simulink model "Simulation_Fahrmodell_v4_straight_line_v1"  (R2023b)
settings: Solver=ode14x  StartTime=0.0  StopTime=500  FixedStep=0.005  RelTol=1e-3
undefined symbols (not defined in the file): bat, cp, cp_Zelle_JpkgK, gb, Ice_derfacLoadDecrease_MAP, Ice_derfacLoadIncrease_MAP, Ice_n_axis, Ice_relLoadMax_CUR_n, Ice_relLoadMax_CUR_val, Ice_rl_axis_norm, P4, P4_DM, pt, seconds, SKO_STREET_CHAL, SKO_WHEEL_TYP_CHAL, slip_pacejka, T_init_degC, Track, TT_sliced, use_turbo_model, v_Fzg_init_kmph, veh
libraries: nesl_utility x15, fl_lib x9, simulink x4
(part 4 of 7)

== system Simulation_Fahrmodell_v4_straight_line_v1/Vehicle Dynamics Model /Drivetrain/GETRIEBE auswahl VK, EV/Transmission Selector1/ICE Multi-Speed/Simulation Doppelkupplung (Gangwechsel ohne Zugkraftunterbrechung) orig2 ==
  i_GET : Inport
  GANG : Inport  Port=2
  Add : Sum
  Berechne prozentuale Zeit bis zum 0.3s : Product  Inputs=*/
  Berechne Negation der prozentualen Zeit : Sum  Inputs=+-
  Berechnung Zeit : Integrator  ExternalReset=falling
  Clock : Clock
  Constant : Constant  Value=0
  Constant1 : Constant
  Constant2 : Constant  Value=0
  Delay : Delay  DelayLength=1  InitialConditionSource=Input port  InitialCondition=1
      settings: InputPortMap=u0,p4
  Display5 : Display
  Gang davor * proz. Zeit : Product
  Gang neu * proz. Zeit : Product
  MATLAB Function : MATLAB Function  TreatAsAtomicUnit=on
  "Nach Trigger -> 0.3s auf True halten" : MATLAB Function  TreatAsAtomicUnit=on
  "Prozentuale Zeit = 0 -> kein Gangwechsel" : RelationalOperator  Operator===  OutDataTypeStr=boolean  RndMeth=Simplest  InputSameDT=off
  Scope : Scope  NumInputPorts=2
  Scope1 : Scope
  Scope2 : Scope  NumInputPorts=2
  Switch : Switch  Criteria=u2 > Threshold  SaturateOnIntegerOverflow=off  InputSameDT=off
  Time to hold (s) : Constant  Value=0.15
  Vgl. Gang aktuell und Gang davor : RelationalOperator  Operator=~=  OutDataTypeStr=boolean  RndMeth=Simplest  InputSameDT=off
  Vorheriger Wert : Subsystem  Commented=on
  Zappeln vermeiden : Delay  DelayLength=1  InitialConditionSource=Input port
      settings: InputPortMap=u0,p4
  i_GET DKG : Outport
  wires:
  "Prozentuale Zeit = 0 -> kein Gangwechsel"/1 -> Switch/2
  Switch/1 -> i_GET DKG/1
  Constant/1 -> "Prozentuale Zeit = 0 -> kein Gangwechsel"/2
  Gang davor * proz. Zeit/1 -> Add/1
  Berechnung Zeit/1 -> Berechne prozentuale Zeit bis zum 0.3s/1
  Berechne Negation der prozentualen Zeit/1 -> Gang davor * proz. Zeit/2
  Add/1 -> Switch/3
  Vgl. Gang aktuell und Gang davor/1 -> "Nach Trigger -> 0.3s auf True halten"/2(enableSignal)
  Delay/1 -> Vgl. Gang aktuell und Gang davor/2
  Constant1/1 -> Berechne Negation der prozentualen Zeit/1
  "Nach Trigger -> 0.3s auf True halten"/1(out) -> Display5/1, Berechnung Zeit/1, Berechnung Zeit/2, Scope/2  "Output"
  MATLAB Function/1(y) -> Scope2/1, Gang davor * proz. Zeit/1
  Gang neu * proz. Zeit/1 -> Add/2
  Clock/1 -> "Nach Trigger -> 0.3s auf True halten"/1(clkTime)
  Zappeln vermeiden/1 -> Switch/1
  Berechne prozentuale Zeit bis zum 0.3s/1 -> Scope1/1, Gang neu * proz. Zeit/2, "Prozentuale Zeit = 0 -> kein Gangwechsel"/1, Berechne Negation der prozentualen Zeit/2
  i_GET/1 -> MATLAB Function/1(i_GET), Gang neu * proz. Zeit/1, Zappeln vermeiden/2, Zappeln vermeiden/1, Scope2/2
  Time to hold (s)/1 -> "Nach Trigger -> 0.3s auf True halten"/3(timeWait), Berechne prozentuale Zeit bis zum 0.3s/2
  GANG/1 -> Delay/2, Scope/1, Vgl. Gang aktuell und Gang davor/1, Delay/1
  Constant2/1 -> MATLAB Function/2(reset)

== system Simulation_Fahrmodell_v4_straight_line_v1/Vehicle Dynamics Model /Drivetrain/GETRIEBE auswahl VK, EV/Transmission Selector1/ICE Multi-Speed/Subsystem1 ==
  Current rpm : Inport
  upshift : Inport  Port=2
  downshift : Inport  Port=3
  Begrenzung Gang1 : Saturate  UpperLimit=10  LowerLimit=1
  Constant : Constant  Value=0.005
  Constant3 : Constant  Value=gb.shiftDelay
  Delay Init = 1st Gear : Delay  DelayLength=1  InitialCondition=1
  "Desired Gear " : Subsystem
  "Locktime Bypass Conditions " : Subsystem
  Relational Operator3 : RelationalOperator  Operator=<=  OutDataTypeStr=boolean  RndMeth=Simplest  InputSameDT=off
  Relational Operator4 : RelationalOperator  OutDataTypeStr=boolean  RndMeth=Simplest  InputSameDT=off
  Scope : Scope  NumInputPorts=2
  Scope1 : Scope  NumInputPorts=2
  "Shift Delay and Clutch Disengagement " : MATLAB Function  TreatAsAtomicUnit=on
  gear latch : MATLAB Function  TreatAsAtomicUnit=on
  Current_Gear : Outport
  tag scope: Clutch_Engaged=global
  wires:
  Relational Operator4/1 -> "Desired Gear "/2(Upshift_Signal), gear latch/1(upshift)  "u"
  "Shift Delay and Clutch Disengagement "/1(currentGear) -> Scope1/1, Begrenzung Gang1/1  "Normal"
  Constant/1 -> "Shift Delay and Clutch Disengagement "/2(dt)
  Begrenzung Gang1/1 -> Current_Gear/1, Delay Init = 1st Gear/1  "Normal"
  "Shift Delay and Clutch Disengagement "/2(clutchEngaged) -> [Clutch_Engaged], Scope1/2  "clutchEngaged"
  Constant3/1 -> "Shift Delay and Clutch Disengagement "/3(shiftDelay)
  Relational Operator3/1 -> gear latch/2(downshift), "Desired Gear "/4(Downshift_Signal)  "d"
  Current rpm/1 -> Relational Operator3/1, "Locktime Bypass Conditions "/2(Current Rpm), Relational Operator4/1  "Current Rpm"
  upshift/1 -> Relational Operator4/2, "Locktime Bypass Conditions "/1(Gear upshift Rpm)  "Gear upshift Rpm"
  downshift/1 -> Relational Operator3/2, "Locktime Bypass Conditions "/3(Gear downshift Rpm)  "Gear downshift Rpm"
  "Locktime Bypass Conditions "/1(cmd_Bypass_Lock_time) -> gear latch/3(cmd_Bypass_Lock_time)  "bypass"
  Delay Init = 1st Gear/1 -> Scope/1, "Desired Gear "/1(Current Gear)
  gear latch/1(shift_cmd) -> "Desired Gear "/3(cmd)  "cmd"
  "Desired Gear "/1(desiredGear) -> Scope/2, "Shift Delay and Clutch Disengagement "/1(desiredGear)

== system Simulation_Fahrmodell_v4_straight_line_v1/Vehicle Dynamics Model /Drivetrain/Primary and Secondary Axle Powertrain Selector/Primary Axle Powertrain Selector/Electric Drive/Variant Subsystem ==
  note: 1) Add Subsystem or Model blocks as valid variant choices.
      | 2) You cannot connect blocks at this level. At simulation, connectivity is automatically
      | determined, based on the active variant and port name matching.
  i_ges : Inport
  Regelfaktor1 : Inport  Port=2
  iAG : Inport  Port=3
  n_mot_Upmin : Inport  Port=4
  Torque_sh : Inport  Port=5
  EV Dual Motor : Subsystem  VariantControl=pt.E1 == 1
  EV Single Motor : Subsystem  VariantControl=pt.E0 == 1
  "M_Nm GET VKM, EM, P1, P2, P3" : Outport

== system Simulation_Fahrmodell_v4_straight_line_v1/Vehicle Dynamics Model /Drivetrain/Primary and Secondary Axle Powertrain Selector/Primary Axle Powertrain Selector/Hybrid Drive/Begrenzung Getriebeeingang Drehmoment und Leistung ==
  n_Upmin : Inport
  M_Nm : Inport  Port=2
  Abs : Abs  SaturateOnIntegerOverflow=off
  Begrenzung Drehmoment : Constant  Value=999999
  Begrenzung Leistung : Constant  Value=999999
  Constant : Constant
  Constant1 : Constant  Value=2*pi/60/1000
  Divide : Product  Inputs=*//
  Gain : Gain  Gain=-1
  Max1 : MinMax  Inputs=3
  Max2 : MinMax  Function=max  Inputs=2
  Switch : Switch  Criteria=u2 > Threshold  SaturateOnIntegerOverflow=off  InputSameDT=off
  Switch1 : Switch  Criteria=u2 > Threshold  SaturateOnIntegerOverflow=off  InputSameDT=off
  M_begr_Nm : Outport
  wires:
  n_Upmin/1 -> Max2/1
  Begrenzung Leistung/1 -> Divide/1  "P_begr_Nm"
  Constant1/1 -> Divide/2
  Constant/1 -> Max2/2
  Max2/1 -> Divide/3
  Divide/1 -> Max1/3
  Begrenzung Drehmoment/1 -> Max1/2
  Switch/1 -> Max1/1
  Switch1/1 -> M_begr_Nm/1
  M_Nm/1 -> Switch1/2, Switch/2, Switch/1, Abs/1
  Abs/1 -> Switch/3
  Max1/1 -> Gain/1, Switch1/1
  Gain/1 -> Switch1/3

== system Simulation_Fahrmodell_v4_straight_line_v1/Vehicle Dynamics Model /Drivetrain/Primary and Secondary Axle Powertrain Selector/Primary Axle Powertrain Selector/Hybrid Drive/ICE ==
  n_Upmin IN : Inport
  Torque_ICE_sh : Inport  Port=2
  GANG : Inport  Port=3
  Berechnung Leistung 1 : Subsystem
  Berechnung Leistung 4 : Subsystem
  Constant : Constant  Value=-25
  Launch Control Drehzahl im 1. Gang : Constant  Value=3000
  "Launch Control logik: 1. Gang, Drehzahl \"halten\"" : Subsystem
  "Max. Kennlinie VKM, Fahren" : Lookup_n-D  NumberOfTableDimensions=1  BreakpointsForDimension1=cp.speed_breakpoints_ICE  Table=cp.torque_values_ICE  ExtrapMethod=Clip  UseLastTableValue=on  InternalRulePriority=Speed  RndMeth=Simplest
  Min : MinMax  Inputs=2
  Saturation : Saturate  UpperLimit=1000  LowerLimit=0
  Scope : Scope  NumInputPorts=3
  Scope1 : Scope  NumInputPorts=2
  Turbo Lag (Beta) : Subsystem  Commented=on
  VKM_M_Nm_Fahren : Outport
  P_max_VKM_kW : Outport  Port=2
  P_min_VKM_kW : Outport  Port=3
  VKM_M_Nm_Reku : Outport  Port=4
  tag scope: tq_sh_ICE_max=global
  wires:
  "Max. Kennlinie VKM, Fahren"/1 -> Scope/3, [tq_sh_ICE_max], Scope1/1, Min/1  "Torque_ICE_Limit"
  Torque_ICE_sh/1 -> Saturation/1
  Constant/1 -> VKM_M_Nm_Reku/1, Berechnung Leistung 4/2(M_Nm)  "VKM_M_Nm_Reku"
  Saturation/1 -> Min/2
  Min/1 -> Scope1/2, VKM_M_Nm_Fahren/1, Berechnung Leistung 1/2(M_Nm)  "VKM_M_Nm_Fahren"
  Berechnung Leistung 1/1(P_kW) -> P_max_VKM_kW/1  "P_ICE_Limit"
  Berechnung Leistung 4/1(P_kW) -> P_min_VKM_kW/1
  "Launch Control logik: 1. Gang, Drehzahl \"halten\""/1(n_mot_lookup (Launch Control)) -> Scope/2, "Max. Kennlinie VKM, Fahren"/1, Berechnung Leistung 1/1(n_Upmin), Berechnung Leistung 4/1(n_Upmin)  "n_ICE"
  Launch Control Drehzahl im 1. Gang/1 -> "Launch Control logik: 1. Gang, Drehzahl \"halten\""/1(Launch Control Drehzahl)  "Launch Control  Drehzahl"
  GANG/1 -> "Launch Control logik: 1. Gang, Drehzahl \"halten\""/2(Gang)
  n_Upmin IN/1 -> Scope/1, "Launch Control logik: 1. Gang, Drehzahl \"halten\""/3(Motordrehzahl (1/min))  "Phys. Motordrehzahl [1/min]"

== system Simulation_Fahrmodell_v4_straight_line_v1/Vehicle Dynamics Model /Drivetrain/Primary and Secondary Axle Powertrain Selector/Primary Axle Powertrain Selector/Hybrid Drive/P0 ==
  note: 1) Add Subsystem or Model blocks as valid variant choices.
      | 2) You cannot connect blocks at this level. At simulation, connectivity is automatically
      | determined, based on the active variant and port name matching.
  n_Upmin IN : Inport
  Torque_P0_sh : Inport  Port=2
  P_max_EM_kW : Inport  Port=3
  P_min_EM_kW : Inport  Port=4
  P0 Motor : Subsystem  VariantControl=pt.P0 == 1
  P0 Motor disabled : Subsystem  VariantControl=pt.P0 == 0
  P0_M_Nm_Fahren : Outport
  P_max_EM_P0_kW : Outport  Port=2
  P_min_EM_P0_kW : Outport  Port=3
  P0_M_Nm_Reku : Outport  Port=4

== system Simulation_Fahrmodell_v4_straight_line_v1/Vehicle Dynamics Model /Drivetrain/Primary and Secondary Axle Powertrain Selector/Primary Axle Powertrain Selector/Hybrid Drive/P2 ==
  note: 1) Add Subsystem or Model blocks as valid variant choices.
      | 2) You cannot connect blocks at this level. At simulation, connectivity is automatically
      | determined, based on the active variant and port name matching.
  n_Upmin IN : Inport
  Torque_P2_sh : Inport  Port=2
  P_max_EM_kW : Inport  Port=3
  P_min_EM_kW : Inport  Port=4
  P2 Motor : Subsystem  VariantControl=pt.P2 == 1
  P2 Motor disabled : Subsystem  VariantControl=pt.P2 == 0
  P2_M_Nm_Fahren : Outport
  P2_M_Nm_Reku : Outport  Port=2
  P_max_EM_P2_kW : Outport  Port=3
  P_min_EM_P2_kW : Outport  Port=4

== system Simulation_Fahrmodell_v4_straight_line_v1/Vehicle Dynamics Model /Drivetrain/Primary and Secondary Axle Powertrain Selector/Primary Axle Powertrain Selector/Hybrid Drive/P3 ==
  note: 1) Add Subsystem or Model blocks as valid variant choices.
      | 2) You cannot connect blocks at this level. At simulation, connectivity is automatically
      | determined, based on the active variant and port name matching.
  n_Upmin IN : Inport
  tq_sh_P3_des : Inport  Port=2
  P_max_EM_kW : Inport  Port=3
  P_min_EM_kW : Inport  Port=4
  P3 Motor : Subsystem  VariantControl=pt.P3 == 1
  P3 Motor disabled : Subsystem  VariantControl=pt.P3 == 0
  P3_M_Nm_Drive : Outport
  P3_M_Nm_Recu : Outport  Port=2
  P_max_EM_P3_kW : Outport  Port=3
  P_min_EM_P3_kW : Outport  Port=4

== system Simulation_Fahrmodell_v4_straight_line_v1/Vehicle Dynamics Model /Drivetrain/Primary and Secondary Axle Powertrain Selector/Primary Axle Powertrain Selector/Hybrid Drive/Recuperation Limit ==
  Torque_Recu_In : Inport
  Constant : Constant  Value=0
  Gain5 : Gain  Gain=100
  Recuperation Limit : Constant  Value=bat.SOC_Recup_Limit
  Relational Operator2 : RelationalOperator  Operator=<  OutDataTypeStr=boolean  RndMeth=Simplest  InputSameDT=off
  Switch2 : Switch  Criteria=u2 > Threshold  SaturateOnIntegerOverflow=off  InputSameDT=off
  Torque_Recu_Out : Outport
  wires:
  Constant/1 -> Switch2/3
  [SOC] -> Relational Operator2/1
  Recuperation Limit/1 -> Gain5/1
  Relational Operator2/1 -> Switch2/2
  Torque_Recu_In/1 -> Switch2/1
  Switch2/1 -> Torque_Recu_Out/1
  Gain5/1 -> Relational Operator2/2

== system Simulation_Fahrmodell_v4_straight_line_v1/Vehicle Dynamics Model /Drivetrain/Primary and Secondary Axle Powertrain Selector/Primary Axle Powertrain Selector/Hybrid Drive/Recuperation Limit1 ==
  Torque_Recu_In : Inport
  Constant : Constant  Value=0
  Gain5 : Gain  Gain=100
  Recuperation Limit : Constant  Value=bat.SOC_Recup_Limit
  Relational Operator2 : RelationalOperator  Operator=<  OutDataTypeStr=boolean  RndMeth=Simplest  InputSameDT=off
  Switch2 : Switch  Criteria=u2 > Threshold  SaturateOnIntegerOverflow=off  InputSameDT=off
  Torque_Recu_Out : Outport
  wires:
  Constant/1 -> Switch2/3
  [SOC] -> Relational Operator2/1
  Recuperation Limit/1 -> Gain5/1
  Relational Operator2/1 -> Switch2/2
  Torque_Recu_In/1 -> Switch2/1
  Switch2/1 -> Torque_Recu_Out/1
  Gain5/1 -> Relational Operator2/2

== system Simulation_Fahrmodell_v4_straight_line_v1/Vehicle Dynamics Model /Drivetrain/Primary and Secondary Axle Powertrain Selector/Primary Axle Powertrain Selector/Hybrid Drive/Shifting Power Cut ==
  In1 : Inport
  Constant : Constant  Value=100
  Switch2 : Switch  Criteria=u2 > Threshold  SaturateOnIntegerOverflow=off  InputSameDT=off
  Out1 : Outport
  wires:
  Constant/1 -> Switch2/3
  In1/1 -> Switch2/1
  Switch2/1 -> Out1/1
  [Clutch_Engaged] -> Switch2/2

== system Simulation_Fahrmodell_v4_straight_line_v1/Vehicle Dynamics Model /Drivetrain/Primary and Secondary Axle Powertrain Selector/Primary Axle Powertrain Selector/Hybrid Drive/Shifting Power Cut1 ==
  In1 : Inport
  Constant : Constant  Value=-100
  Switch2 : Switch  Criteria=u2 > Threshold  SaturateOnIntegerOverflow=off  InputSameDT=off
  Out1 : Outport
  wires:
  [Clutch_Engaged] -> Switch2/2
  Switch2/1 -> Out1/1
  In1/1 -> Switch2/1
  Constant/1 -> Switch2/3

== system Simulation_Fahrmodell_v4_straight_line_v1/Vehicle Dynamics Model /Drivetrain/Primary and Secondary Axle Powertrain Selector/Primary Axle Powertrain Selector/Hybrid Drive/Wirkungsgrad Antriebsstrang ==
  M_Nm IN : Inport
  Constant1 : Constant  Value=0.92
  Fahren : Product
  Reku : Product  Inputs=*/
  Switch1 : Switch  Criteria=u2 > Threshold  SaturateOnIntegerOverflow=off  InputSameDT=off
  M_Nm OUT : Outport
  wires:
  Constant1/1 -> Reku/2, Fahren/2
  M_Nm IN/1 -> Switch1/2, Reku/1, Fahren/1
  Reku/1 -> Switch1/3
  Switch1/1 -> M_Nm OUT/1
  Fahren/1 -> Switch1/1

== system Simulation_Fahrmodell_v4_straight_line_v1/Vehicle Dynamics Model /Drivetrain/Primary and Secondary Axle Powertrain Selector/Secondary Axle Powertrain Selector/Auswahl P4, P4_Dual-Motor/No Secondary Axle ==
  n_mot_Upmin : Inport
  Regelfaktor1 : Inport  Port=2
  iAG : Inport  Port=3
  i_ges : Inport  Port=4
  Torque_sh : Inport  Port=5
  Constant : Constant  Value=0
  Terminator{,1..4} (5 alike) : Terminator
  M_Nm GET P4 : Outport
  wires:
  Constant/1 -> M_Nm GET P4/1
  i_ges/1 -> Terminator/1
  iAG/1 -> Terminator1/1
  Regelfaktor1/1 -> Terminator2/1
  n_mot_Upmin/1 -> Terminator3/1
  Torque_sh/1 -> Terminator4/1

== system Simulation_Fahrmodell_v4_straight_line_v1/Vehicle Dynamics Model /Drivetrain/Primary and Secondary Axle Powertrain Selector/Secondary Axle Powertrain Selector/Auswahl P4, P4_Dual-Motor/P4 // E2 Single Motor ==
  n_mot_Upmin : Inport
  Regelfaktor1 : Inport  Port=2
  iAG : Inport  Port=3
  i_ges : Inport  Port=4
  Torque_sh : Inport  Port=5
  1-D Lookup Table1 : Lookup_n-D  NumberOfTableDimensions=1  BreakpointsForDimension1=cp.speed_breakpoints_P4  Table=cp.torque_values_P4  InternalRulePriority=Speed  RndMeth=Simplest
  AG Übersetzung : Product
  Battery and Operating Strategy Limitation (Drive) : Subsystem
  Battery and Operating Strategy Limitation (Recuperation) : Subsystem
  Bus Selector : BusSelector  OutputSignals=tq_sh_P4_des
  Constant : Constant  Value=gb.i_ges_P4
  Constant1 : Constant  Value=gb.i_ges_P4
  Constant5 : Constant  Value=0
  Divide : Product  Inputs=*/
  Gain : Gain  Gain=-1
  Min : MinMax  Inputs=2
  Power Calculation : Subsystem
  "Power Calculation " : Subsystem
  Product : Product
  Relational Operator1 : RelationalOperator  OutDataTypeStr=boolean  RndMeth=Simplest  InputSameDT=off
  Saturation : Saturate  UpperLimit=inf  LowerLimit=0
  Saturation1 : Saturate  UpperLimit=inf  LowerLimit=1
  Smoothing Logic sanfterer Übergang1 : TransferFcn  Denominator=[0.005 1]
  Switch1 : Switch  Criteria=u2 > Threshold  SaturateOnIntegerOverflow=off  InputSameDT=off
  Terminator : Terminator
  M_Nm GET P4 : Outport
  tag scope: P_max_EM_P4_kW=global, P_min_EM_P4_kW=global, tq_sh_P4_max=global
  wires:
  Regelfaktor1/1 -> Relational Operator1/1  "Regelfaktor1"
  Smoothing Logic sanfterer Übergang1/1 -> AG Übersetzung/2
  Relational Operator1/1 -> Switch1/2
  Constant5/1 -> Relational Operator1/2
  Switch1/1 -> Smoothing Logic sanfterer Übergang1/1  "Gesamtmoment motorseitig"
  AG Übersetzung/1 -> M_Nm GET P4/1
  Constant/1 -> AG Übersetzung/1
  iAG/1 -> Terminator/1  "iAG"
  i_ges/1 -> Saturation1/1
  Power Calculation/1(P_kW) -> [P_max_EM_P4_kW]  "P_max_EM_P4_kW"
  Bus Selector/1 -> Saturation/1  "<tq_sh_P4_des>"
  Product/1 -> Battery and Operating Strategy Limitation (Recuperation)/1(Motordrehzahl (1/min)), Battery and Operating Strategy Limitation (Drive)/1(Motordrehzahl (1/min)), 1-D Lookup Table1/1  "Motordrehzahl (1/min)"
  Saturation/1 -> Min/2
  "Power Calculation "/1(P_kW) -> [P_min_EM_P4_kW]  "P_min_EM_P4_kW"
  1-D Lookup Table1/1 -> Gain/1, [tq_sh_P4_max], Min/1
  Torque_sh/1 -> Bus Selector/1
  n_mot_Upmin/1 -> Divide/1  "Motordrehzahl (1/min)"
  Divide/1 -> Product/1  "Motordrehzahl (1/min)"
  Constant1/1 -> Product/2
  Saturation1/1 -> Divide/2
  Battery and Operating Strategy Limitation (Drive)/2(tq_sh_P4_bat_limted) -> Switch1/1, Power Calculation/2(tq_sh_P4_bat_limted)
  Min/1 -> Battery and Operating Strategy Limitation (Drive)/2(Torque_Drive_In)
  [P_max_EM_kW] -> Battery and Operating Strategy Limitation (Drive)/3(P_max_EV_kW)  "P_max_EM_kW"
  Battery and Operating Strategy Limitation (Drive)/1(n_Upmin OUT) -> Power Calculation/1(n_Upmin)
  Battery and Operating Strategy Limitation (Recuperation)/2(tq_sh_P4_bat_limted_recu) -> Switch1/3, "Power Calculation "/2(tq_sh_P4_bat_limted_recu)
  Gain/1 -> Battery and Operating Strategy Limitation (Recuperation)/2(Torque_Recu_In)
  [P_min_EM_kW] -> Battery and Operating Strategy Limitation (Recuperation)/3(P_min_EV_kW)  "P_min_EM_kW"
  Battery and Operating Strategy Limitation (Recuperation)/1(n_Upmin OUT) -> "Power Calculation "/1(n_Upmin)

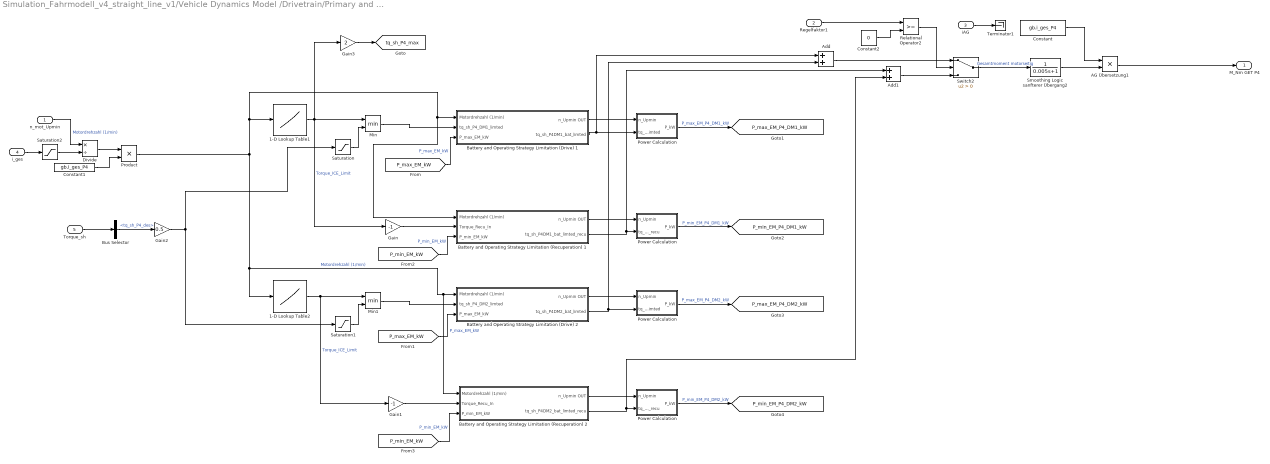
== system Simulation_Fahrmodell_v4_straight_line_v1/Vehicle Dynamics Model /Drivetrain/Primary and Secondary Axle Powertrain Selector/Secondary Axle Powertrain Selector/Auswahl P4, P4_Dual-Motor/P4 // E3 // E4 Dual Motor ==
  n_mot_Upmin : Inport
  Regelfaktor1 : Inport  Port=2
  iAG : Inport  Port=3
  i_ges : Inport  Port=4
  Torque_sh : Inport  Port=5
  1-D Lookup Table1 : Lookup_n-D  NumberOfTableDimensions=1  BreakpointsForDimension1=cp.speed_breakpoints_P4  Table=cp.torque_values_P4  InternalRulePriority=Speed  RndMeth=Simplest
  1-D Lookup Table2 : Lookup_n-D  NumberOfTableDimensions=1  BreakpointsForDimension1=cp.speed_breakpoints_P4  Table=cp.torque_values_P4  InternalRulePriority=Speed  RndMeth=Simplest
  AG Übersetzung1 : Product
  Add : Sum
  Add1 : Sum
  Battery and Operating Strategy Limitation (Drive) 1 : Subsystem
  Battery and Operating Strategy Limitation (Drive) 2 : Subsystem
  Battery and Operating Strategy Limitation (Recuperation) 1 : Subsystem
  Battery and Operating Strategy Limitation (Recuperation) 2 : Subsystem
  Bus Selector : BusSelector  OutputSignals=tq_sh_P4_des
  Constant : Constant  Value=gb.i_ges_P4
  Constant1 : Constant  Value=gb.i_ges_P4
  Constant2 : Constant  Value=0
  Divide : Product  Inputs=*/
  Gain : Gain  Gain=-1
  Gain1 : Gain  Gain=-1
  Gain2 : Gain  Gain=0.5
  Gain3 : Gain  Gain=2
  Min : MinMax  Inputs=2
  Min1 : MinMax  Inputs=2
  "Power Calculation " : Subsystem
  "Power Calculation   " : Subsystem
  "Power Calculation    " : Subsystem
  "Power Calculation     " : Subsystem
  Product : Product
  Relational Operator2 : RelationalOperator  OutDataTypeStr=boolean  RndMeth=Simplest  InputSameDT=off
  Saturation : Saturate  UpperLimit=inf  LowerLimit=0
  Saturation1 : Saturate  UpperLimit=inf  LowerLimit=0
  Saturation2 : Saturate  UpperLimit=inf  LowerLimit=1
  Smoothing Logic sanfterer Übergang2 : TransferFcn  Denominator=[0.005 1]
  Switch2 : Switch  Criteria=u2 > Threshold  SaturateOnIntegerOverflow=off  InputSameDT=off
  Terminator1 : Terminator
  M_Nm GET P4 : Outport
  tag scope: P_max_EM_P4_DM1_kW=global, P_max_EM_P4_DM2_kW=global, P_min_EM_P4_DM1_kW=global, P_min_EM_P4_DM2_kW=global, tq_sh_P4_max=global
  wires:
  Bus Selector/1 -> Gain2/1  "<tq_sh_P4_des>"
  "Power Calculation    "/1(P_kW) -> [P_min_EM_P4_DM1_kW]  "P_min_EM_P4_DM1_kW"
  Torque_sh/1 -> Bus Selector/1
  "Power Calculation     "/1(P_kW) -> [P_max_EM_P4_DM1_kW]  "P_max_EM_P4_DM1_kW"
  1-D Lookup Table1/1 -> Gain3/1, Min/1, Gain/1  "Torque_ICE_Limit"
  Saturation/1 -> Min/2
  "Power Calculation "/1(P_kW) -> [P_min_EM_P4_DM2_kW]  "P_min_EM_P4_DM2_kW"
  "Power Calculation   "/1(P_kW) -> [P_max_EM_P4_DM2_kW]  "P_max_EM_P4_DM2_kW"
  1-D Lookup Table2/1 -> Gain1/1, Min1/1  "Torque_ICE_Limit"
  Saturation1/1 -> Min1/2
  AG Übersetzung1/1 -> M_Nm GET P4/1
  Constant/1 -> AG Übersetzung1/1
  Switch2/1 -> Smoothing Logic sanfterer Übergang2/1  "Gesamtmoment motorseitig"
  iAG/1 -> Terminator1/1
  Relational Operator2/1 -> Switch2/2
  Regelfaktor1/1 -> Relational Operator2/1
  Add1/1 -> Switch2/3
  Constant2/1 -> Relational Operator2/2
  Add/1 -> Switch2/1
  Smoothing Logic sanfterer Übergang2/1 -> AG Übersetzung1/2
  Gain2/1 -> Saturation/1, Saturation1/1
  n_mot_Upmin/1 -> Divide/1  "Motordrehzahl (1/min)"
  i_ges/1 -> Saturation2/1
  Divide/1 -> Product/1
  Constant1/1 -> Product/2
  Product/1 -> Battery and Operating Strategy Limitation (Recuperation) 1/1(Motordrehzahl (1/min)), Battery and Operating Strategy Limitation (Drive) 1/1(Motordrehzahl (1/min)), 1-D Lookup Table1/1, 1-D Lookup Table2/1, Battery and Operating Strategy Limitation (Recuperation) 2/1(Motordrehzahl (1/min)), Battery and Operating Strategy Limitation (Drive) 2/1(Motordrehzahl (1/min))  "Motordrehzahl (1/min)"
  Saturation2/1 -> Divide/2
  Gain3/1 -> [tq_sh_P4_max]
  Battery and Operating Strategy Limitation (Drive) 1/2(tq_sh_P4DM1_bat_limted) -> Add/1, "Power Calculation     "/2(tq_sh_P4DM1_bat_limted)
  Min/1 -> Battery and Operating Strategy Limitation (Drive) 1/2(tq_sh_P4_DM1_limted)
  [P_max_EM_kW] -> Battery and Operating Strategy Limitation (Drive) 1/3(P_max_EM_kW)  "P_max_EM_kW"
  Battery and Operating Strategy Limitation (Drive) 1/1(n_Upmin OUT) -> "Power Calculation     "/1(n_Upmin)
  Battery and Operating Strategy Limitation (Recuperation) 1/2(tq_sh_P4DM1_bat_limted_recu) -> Add1/1, "Power Calculation    "/2(tq_sh_P4DM1_bat_limted_recu)
  Gain/1 -> Battery and Operating Strategy Limitation (Recuperation) 1/2(Torque_Recu_In)
  [P_min_EM_kW] -> Battery and Operating Strategy Limitation (Recuperation) 1/3(P_min_EM_kW)  "P_min_EM_kW"
  Battery and Operating Strategy Limitation (Recuperation) 1/1(n_Upmin OUT) -> "Power Calculation    "/1(n_Upmin)
  Battery and Operating Strategy Limitation (Drive) 2/2(tq_sh_P4DM2_bat_limted) -> Add/2, "Power Calculation   "/2(tq_sh_P4DM2_bat_limted)
  Min1/1 -> Battery and Operating Strategy Limitation (Drive) 2/2(tq_sh_P4_DM2_limted)
  [P_max_EM_kW] -> Battery and Operating Strategy Limitation (Drive) 2/3(P_max_EM_kW)  "P_max_EM_kW"
  Battery and Operating Strategy Limitation (Drive) 2/1(n_Upmin OUT) -> "Power Calculation   "/1(n_Upmin)
  Battery and Operating Strategy Limitation (Recuperation) 2/2(tq_sh_P4DM2_bat_limted_recu) -> Add1/2, "Power Calculation "/2(tq_sh_P4DM2_bat_limted_recu)
  Gain1/1 -> Battery and Operating Strategy Limitation (Recuperation) 2/2(Torque_Recu_In)
  [P_min_EM_kW] -> Battery and Operating Strategy Limitation (Recuperation) 2/3(P_min_EM_kW)  "P_min_EM_kW"
  Battery and Operating Strategy Limitation (Recuperation) 2/1(n_Upmin OUT) -> "Power Calculation "/1(n_Upmin)

== system Simulation_Fahrmodell_v4_straight_line_v1/Vehicle Dynamics Model /Drivetrain/GETRIEBE auswahl VK, EV/Transmission Selector1/ICE Multi-Speed/Simulation Doppelkupplung (Gangwechsel ohne Zugkraftunterbrechung) orig2/Vorheriger Wert ==
  In1 : Inport
  In2 : Inport  Port=2
  Delay : Delay  DelayLength=1  InitialConditionSource=Input port
      settings: InputPortMap=u0,p4
  Memory : Memory
  Relational Operator : RelationalOperator  Operator=~=  OutDataTypeStr=boolean  RndMeth=Simplest  InputSameDT=off
  Switch1 : Switch  Criteria=u2 > Threshold  SaturateOnIntegerOverflow=off  InputSameDT=off
  Out1 : Outport
  wires:
  Switch1/1 -> Memory/1, Out1/1
  Relational Operator/1 -> Switch1/2
  Delay/1 -> Relational Operator/2, Switch1/1
  In1/1 -> Relational Operator/1, Delay/2, Delay/1
  Memory/1 -> Switch1/3

== system Simulation_Fahrmodell_v4_straight_line_v1/Vehicle Dynamics Model /Drivetrain/GETRIEBE auswahl VK, EV/Transmission Selector1/ICE Multi-Speed/Subsystem1/Desired Gear  ==
  Current Gear : Inport
  Upshift_Signal : Inport  Port=2
  cmd : Inport  Port=3
  Downshift_Signal : Inport  Port=4
  Add : Sum
  Add1 : Sum  Inputs=+-
  Begrenzung Gang : Saturate  UpperLimit=gb.No_Gears  LowerLimit=1
  Constant1 : Constant
  Constant2 : Constant
  Constant6 : Constant  Value=0
  Relational Operator1 : RelationalOperator  Operator===  OutDataTypeStr=boolean  RndMeth=Simplest  InputSameDT=off
  Switch{1,3..5} (4 alike) : Switch  Criteria=u2 > Threshold  SaturateOnIntegerOverflow=off  InputSameDT=off
  Unit Delay Init = 1st Gear : UnitDelay  InitialCondition=1  SampleTime=0.005
  desiredGear : Outport
  wires:
  Add1/1 -> Switch4/1
  Current Gear/1 -> Switch1/1, Add1/1, Switch4/3, Switch3/3, Add/1
  Switch1/1 -> Begrenzung Gang/1  "Current_Gear"
  Constant1/1 -> Add/2
  Add/1 -> Switch3/1
  Upshift_Signal/1 -> Switch3/2
  Switch4/1 -> Switch5/3
  cmd/1 -> Switch5/2, Relational Operator1/1
  Switch3/1 -> Switch5/1
  Relational Operator1/1 -> Switch1/2
  Unit Delay Init = 1st Gear/1 -> desiredGear/1
  Switch5/1 -> Switch1/3  "Current_Gear"
  Constant6/1 -> Relational Operator1/2
  Constant2/1 -> Add1/2
  Begrenzung Gang/1 -> Unit Delay Init = 1st Gear/1  "Normal"
  Downshift_Signal/1 -> Switch4/2

== system Simulation_Fahrmodell_v4_straight_line_v1/Vehicle Dynamics Model /Drivetrain/GETRIEBE auswahl VK, EV/Transmission Selector1/ICE Multi-Speed/Subsystem1/Locktime Bypass Conditions  ==
  note: FOR DOWNSHIFT
  note: FOR UPSHIFT
  Gear upshift Rpm : Inport
  Current Rpm : Inport  Port=2
  Gear downshift Rpm : Inport  Port=3
  AND : Logic  IconShape=distinctive  AllPortsSameDT=off  OutDataTypeStr=boolean
  AND1 : Logic  IconShape=distinctive  AllPortsSameDT=off  OutDataTypeStr=boolean
  AND2 : Logic  IconShape=distinctive  AllPortsSameDT=off  OutDataTypeStr=boolean
  Constant{4..5,7..8} (4 alike) : Constant  Value=0
  OR : Logic  Operator=OR  IconShape=distinctive  AllPortsSameDT=off  OutDataTypeStr=boolean
  OR1 : Logic  Operator=OR  IconShape=distinctive  AllPortsSameDT=off  OutDataTypeStr=boolean
  Relational Operator2 : RelationalOperator  Operator=>  OutDataTypeStr=boolean  RndMeth=Simplest  InputSameDT=off
  Relational Operator5 : RelationalOperator  Operator=<=  OutDataTypeStr=boolean  RndMeth=Simplest  InputSameDT=off
  Relational Operator6 : RelationalOperator  Operator=<=  OutDataTypeStr=boolean  RndMeth=Simplest  InputSameDT=off
  Relational Operator7 : RelationalOperator  OutDataTypeStr=boolean  RndMeth=Simplest  InputSameDT=off
  Relational Operator8 : RelationalOperator  Operator=>  OutDataTypeStr=boolean  RndMeth=Simplest  InputSameDT=off
  Relational Operator9 : RelationalOperator  Operator=<=  OutDataTypeStr=boolean  RndMeth=Simplest  InputSameDT=off
  cmd_Bypass_Lock_time : Outport
  wires:
  Constant8/1 -> Relational Operator9/2
  Relational Operator5/1 -> AND1/1
  [Gaspedalposition] -> Relational Operator5/1, Relational Operator8/1, Relational Operator2/1  "Gas Pedal Position"
  Relational Operator7/1 -> AND/2
  Relational Operator2/1 -> AND/1
  Relational Operator6/1 -> AND1/2
  Gear downshift Rpm/1 -> Relational Operator6/2
  Constant4/1 -> Relational Operator2/2
  Current Rpm/1 -> Relational Operator7/1, Relational Operator6/1
  AND1/1 -> OR/1
  Constant7/1 -> Relational Operator8/2
  OR/1 -> OR1/2  "Bypass Lock time"
  AND/1 -> OR1/1  "Bypass Lock time"
  Constant5/1 -> Relational Operator5/2
  AND2/1 -> OR/2
  Relational Operator8/1 -> AND2/1
  Relational Operator9/1 -> AND2/2
  [S_BUS_IST_Profil_a] -> Relational Operator9/1  "Acceleration"
  OR1/1 -> cmd_Bypass_Lock_time/1  "cmd_Bypass_Lock_time"
  Gear upshift Rpm/1 -> Relational Operator7/2

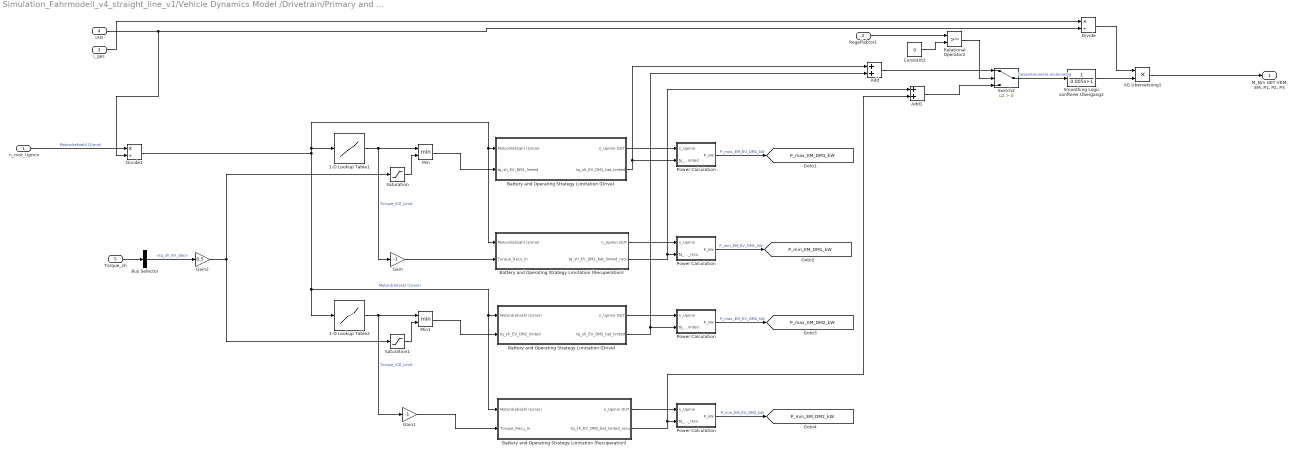
== system Simulation_Fahrmodell_v4_straight_line_v1/Vehicle Dynamics Model /Drivetrain/Primary and Secondary Axle Powertrain Selector/Primary Axle Powertrain Selector/Electric Drive/Variant Subsystem/EV Dual Motor ==
  n_mot_Upmin : Inport
  Regelfaktor1 : Inport  Port=2
  i_ges : Inport  Port=3
  iAG : Inport  Port=4
  Torque_sh : Inport  Port=5
  1-D Lookup Table1 : Lookup_n-D  NumberOfTableDimensions=1  BreakpointsForDimension1=cp.speed_breakpoints_EV  Table=cp.torque_values_EV  InternalRulePriority=Speed  RndMeth=Simplest
  1-D Lookup Table2 : Lookup_n-D  NumberOfTableDimensions=1  BreakpointsForDimension1=cp.speed_breakpoints_EV  Table=cp.torque_values_EV  InternalRulePriority=Speed  RndMeth=Simplest
  AG Übersetzung1 : Product
  Add : Sum
  Add1 : Sum
  Battery and Operating Strategy Limitation (Drive) : Subsystem
  "Battery and Operating Strategy Limitation (Drive) " : Subsystem
  Battery and Operating Strategy Limitation (Recuperation) : Subsystem
  "Battery and Operating Strategy Limitation (Recuperation) " : Subsystem
  Bus Selector : BusSelector  OutputSignals=tq_sh_EV_des
  Constant2 : Constant  Value=0
  Divide : Product  Inputs=*/
  Divide1 : Product  Inputs=*/
  Gain : Gain  Gain=-1
  Gain1 : Gain  Gain=-1
  Gain2 : Gain  Gain=0.5
  Min : MinMax  Inputs=2
  Min1 : MinMax  Inputs=2
  Power Calculation : Subsystem
  "Power Calculation " : Subsystem
  "Power Calculation  " : Subsystem
  "Power Calculation    " : Subsystem
  Relational Operator2 : RelationalOperator  OutDataTypeStr=boolean  RndMeth=Simplest  InputSameDT=off
  Saturation : Saturate  UpperLimit=inf  LowerLimit=0
  Saturation1 : Saturate  UpperLimit=inf  LowerLimit=0
  Smoothing Logic sanfterer Übergang2 : TransferFcn  Denominator=[0.005 1]
  Switch2 : Switch  Criteria=u2 > Threshold  SaturateOnIntegerOverflow=off  InputSameDT=off
  "M_Nm GET VKM, EM, P1, P2, P3" : Outport
  tag scope: P_max_EM_DM1_kW=global, P_max_EM_DM2_kW=global, P_min_EM_DM1_kW=global, P_min_EM_DM2_kW=global
  wires:
  Add1/1 -> Switch2/3
  Add/1 -> Switch2/1
  Switch2/1 -> Smoothing Logic sanfterer Übergang2/1  "Gesamtmoment motorseitig"
  Smoothing Logic sanfterer Übergang2/1 -> AG Übersetzung1/2
  Regelfaktor1/1 -> Relational Operator2/1
  Relational Operator2/1 -> Switch2/2
  AG Übersetzung1/1 -> "M_Nm GET VKM, EM, P1, P2, P3"/1
  Constant2/1 -> Relational Operator2/2
  i_ges/1 -> Divide/1
  iAG/1 -> Divide1/2, Divide/2
  Divide/1 -> AG Übersetzung1/1
  Saturation1/1 -> Min1/2
  "Power Calculation    "/1(P_kW) -> [P_max_EM_DM2_kW]  "P_max_EM_EV_DM2_kW"
  1-D Lookup Table2/1 -> Gain1/1, Min1/1  "Torque_ICE_Limit"
  "Power Calculation  "/1(P_kW) -> [P_min_EM_DM1_kW]  "P_min_EM_EV_DM1_kW"
  "Power Calculation "/1(P_kW) -> [P_max_EM_DM1_kW]  "P_max_EM_EV_DM1_kW"
  Divide1/1 -> 1-D Lookup Table2/1, "Battery and Operating Strategy Limitation (Recuperation) "/1(Motordrehzahl (1/min)), "Battery and Operating Strategy Limitation (Drive) "/1(Motordrehzahl (1/min)), Battery and Operating Strategy Limitation (Recuperation)/1(Motordrehzahl (1/min)), Battery and Operating Strategy Limitation (Drive)/1(Motordrehzahl (1/min)), 1-D Lookup Table1/1  "Motordrehzahl (1/min)"
  Power Calculation/1(P_kW) -> [P_min_EM_DM2_kW]  "P_min_EM_EV_DM2_kW"
  Gain2/1 -> Saturation1/1, Saturation/1
  Saturation/1 -> Min/2
  1-D Lookup Table1/1 -> Gain/1, Min/1  "Torque_ICE_Limit"
  Torque_sh/1 -> Bus Selector/1
  Bus Selector/1 -> Gain2/1  "<tq_sh_EV_des>"
  n_mot_Upmin/1 -> Divide1/1  "Motordrehzahl (1/min)"
  Battery and Operating Strategy Limitation (Drive)/2(tq_sh_EV_DM1_bat_limted) -> Add/1, "Power Calculation "/2(tq_sh_EV_DM1_bat_limted)
  Min/1 -> Battery and Operating Strategy Limitation (Drive)/2(tq_sh_EV_DM1_limted)
  Battery and Operating Strategy Limitation (Drive)/1(n_Upmin OUT) -> "Power Calculation "/1(n_Upmin)
  Battery and Operating Strategy Limitation (Recuperation)/2(tq_sh_EV_DM1_bat_limted_recu) -> Add1/1, "Power Calculation  "/2(tq_sh_EV_DM1_bat_limted_recu)
  Gain/1 -> Battery and Operating Strategy Limitation (Recuperation)/2(Torque_Recu_In)
  Battery and Operating Strategy Limitation (Recuperation)/1(n_Upmin OUT) -> "Power Calculation  "/1(n_Upmin)
  "Battery and Operating Strategy Limitation (Drive) "/2(tq_sh_EV_DM2_bat_limted) -> Add/2, "Power Calculation    "/2(tq_sh_EV_DM2_bat_limted)
  Min1/1 -> "Battery and Operating Strategy Limitation (Drive) "/2(tq_sh_EV_DM2_limted)
  "Battery and Operating Strategy Limitation (Drive) "/1(n_Upmin OUT) -> "Power Calculation    "/1(n_Upmin)
  "Battery and Operating Strategy Limitation (Recuperation) "/2(tq_sh_EV_DM2_bat_limted_recu) -> Add1/2, Power Calculation/2(tq_sh_EV_DM2_bat_limted_recu)
  Gain1/1 -> "Battery and Operating Strategy Limitation (Recuperation) "/2(Torque_Recu_In)
  "Battery and Operating Strategy Limitation (Recuperation) "/1(n_Upmin OUT) -> Power Calculation/1(n_Upmin)

== system Simulation_Fahrmodell_v4_straight_line_v1/Vehicle Dynamics Model /Drivetrain/Primary and Secondary Axle Powertrain Selector/Primary Axle Powertrain Selector/Electric Drive/Variant Subsystem/EV Single Motor ==
  Regelfaktor1 : Inport
  n_mot_Upmin : Inport  Port=2
  i_ges : Inport  Port=3
  iAG : Inport  Port=4
  Torque_sh : Inport  Port=5
  1-D Lookup Table1 : Lookup_n-D  NumberOfTableDimensions=1  BreakpointsForDimension1=cp.speed_breakpoints_EV  Table=cp.torque_values_EV  InternalRulePriority=Speed  RndMeth=Simplest
  Battery and Operating Strategy Limitation (Drive) : Subsystem
  Battery and Operating Strategy Limitation (Recuperation) : Subsystem
  Bus Selector : BusSelector  OutputSignals=tq_sh_EV_des
  Constant7 : Constant  Value=0
  Gain : Gain  Gain=-1
  Min : MinMax  Inputs=2
  Power Calculation : Subsystem
  "Power Calculation " : Subsystem
  Relational Operator2 : RelationalOperator  OutDataTypeStr=boolean  RndMeth=Simplest  InputSameDT=off
  Saturation : Saturate  UpperLimit=inf  LowerLimit=0
  Smoothing Logic sanfterer Übergang2 : TransferFcn  Denominator=[0.005 1]
  Switch2 : Switch  Criteria=u2 > Threshold  SaturateOnIntegerOverflow=off  InputSameDT=off
  Terminator : Terminator
  Wirkungsgrad Antriebsstrang1 : Subsystem
  i_GES Übersetzung : Product
  "M_Nm GET VKM, EM, P1, P2, P3" : Outport
  tag scope: P_max_EM_EV_kW=global, P_min_EM_EV_kW=global
  wires:
  iAG/1 -> Terminator/1
  Constant7/1 -> Relational Operator2/2
  Smoothing Logic sanfterer Übergang2/1 -> i_GES Übersetzung/2
  Switch2/1 -> Smoothing Logic sanfterer Übergang2/1  "Gesamtmoment motorseitig"
  Wirkungsgrad Antriebsstrang1/1(M_Nm OUT) -> "M_Nm GET VKM, EM, P1, P2, P3"/1
  Relational Operator2/1 -> Switch2/2
  Regelfaktor1/1 -> Relational Operator2/1
  i_GES Übersetzung/1 -> Wirkungsgrad Antriebsstrang1/1(M_Nm IN)
  i_ges/1 -> i_GES Übersetzung/1  "i_GES"
  n_mot_Upmin/1 -> Battery and Operating Strategy Limitation (Recuperation)/1(Motordrehzahl (1/min)), Battery and Operating Strategy Limitation (Drive)/1(Motordrehzahl (1/min)), 1-D Lookup Table1/1  "Motordrehzahl (1/min)"
  Power Calculation/1(P_kW) -> [P_max_EM_EV_kW]  "P_max_EM_EV_kW"
  1-D Lookup Table1/1 -> Min/1, Gain/1  "Torque_ICE_Limit"
  Saturation/1 -> Min/2
  Bus Selector/1 -> Saturation/1  "<tq_sh_EV_des>"
  "Power Calculation "/1(P_kW) -> [P_min_EM_EV_kW]  "P_min_EM_EV_kW"
  Torque_sh/1 -> Bus Selector/1
  Battery and Operating Strategy Limitation (Drive)/2(tq_sh_EM_bat_limted) -> Switch2/1, Power Calculation/2(tq_sh_EM_bat_limted)
  Min/1 -> Battery and Operating Strategy Limitation (Drive)/2(tq_sh_EM_limted)  "tq_sh_EM_limted"
  Battery and Operating Strategy Limitation (Drive)/1(n_Upmin OUT) -> Power Calculation/1(n_Upmin)
  Battery and Operating Strategy Limitation (Recuperation)/2(tq_sh_EM_bat_limted_recu) -> Switch2/3, "Power Calculation "/2(tq_sh_EM_bat_limted_recu)
  Gain/1 -> Battery and Operating Strategy Limitation (Recuperation)/2(Torque_Recu_In)
  Battery and Operating Strategy Limitation (Recuperation)/1(n_Upmin OUT) -> "Power Calculation "/1(n_Upmin)

== system Simulation_Fahrmodell_v4_straight_line_v1/Vehicle Dynamics Model /Drivetrain/Primary and Secondary Axle Powertrain Selector/Primary Axle Powertrain Selector/Hybrid Drive/ICE/Berechnung Leistung 1 ==
  n_Upmin : Inport
  M_Nm : Inport  Port=2
  Constant1 : Constant  Value=2*pi/60/1000
  Product : Product  Inputs=3
  P_kW : Outport
  wires:
  Product/1 -> P_kW/1
  n_Upmin/1 -> Product/2
  Constant1/1 -> Product/3
  M_Nm/1 -> Product/1

== system Simulation_Fahrmodell_v4_straight_line_v1/Vehicle Dynamics Model /Drivetrain/Primary and Secondary Axle Powertrain Selector/Primary Axle Powertrain Selector/Hybrid Drive/ICE/Berechnung Leistung 4 ==
  n_Upmin : Inport
  M_Nm : Inport  Port=2
  Constant1 : Constant  Value=2*pi/60/1000
  Product : Product  Inputs=3
  P_kW : Outport
  wires:
  Product/1 -> P_kW/1
  n_Upmin/1 -> Product/2
  Constant1/1 -> Product/3
  M_Nm/1 -> Product/1

== system Simulation_Fahrmodell_v4_straight_line_v1/Vehicle Dynamics Model /Drivetrain/Primary and Secondary Axle Powertrain Selector/Primary Axle Powertrain Selector/Hybrid Drive/ICE/Launch Control logik: 1. Gang, Drehzahl "halten" ==
  Launch Control Drehzahl : Inport
  Gang : Inport  Port=2
  Motordrehzahl (1/min) : Inport  Port=3
  1. Gang : RelationalOperator  Operator===  OutDataTypeStr=boolean  RndMeth=Simplest  InputSameDT=off
  AND : Logic  IconShape=distinctive  AllPortsSameDT=off  OutDataTypeStr=boolean
  Constant1 : Constant
  Switch : Switch  Criteria=u2 > Threshold  SaturateOnIntegerOverflow=off  InputSameDT=off
  n < 3000 U/min : RelationalOperator  Operator=<  OutDataTypeStr=boolean  RndMeth=Simplest  InputSameDT=off
  n_mot_lookup (Launch Control) : Outport
  wires:
  Launch Control Drehzahl/1 -> Switch/1, n < 3000 U/min/2
  1. Gang/1 -> AND/1
  Gang/1 -> 1. Gang/1
  Switch/1 -> n_mot_lookup (Launch Control)/1  "n_mot_lookup (Launch Control)"
  AND/1 -> Switch/2
  Motordrehzahl (1/min)/1 -> n < 3000 U/min/1, Switch/3
  n < 3000 U/min/1 -> AND/2
  Constant1/1 -> 1. Gang/2

== system Simulation_Fahrmodell_v4_straight_line_v1/Vehicle Dynamics Model /Drivetrain/Primary and Secondary Axle Powertrain Selector/Primary Axle Powertrain Selector/Hybrid Drive/ICE/Turbo Lag (Beta) ==
  Torque_ICE_Limit : Inport
  Motordrehzahl (1/min) : Inport  Port=2
  Constant1 : Constant  Value=use_turbo_model
  Product : Product
  Switch : Switch  Criteria=u2 > Threshold  SaturateOnIntegerOverflow=off  InputSameDT=off
  Turbo Lag : Subsystem
  Out1 : Outport
  wires:
  Motordrehzahl (1/min)/1 -> Turbo Lag/1(n_ICE)
  Switch/1 -> Out1/1
  Product/1 -> Switch/1
  Torque_ICE_Limit/1 -> Product/2, Switch/3
  Constant1/1 -> Switch/2
  Turbo Lag/1(rl) -> Product/1
  [Gaspedalposition] -> Turbo Lag/2(rl_des)

== system Simulation_Fahrmodell_v4_straight_line_v1/Vehicle Dynamics Model /Drivetrain/Primary and Secondary Axle Powertrain Selector/Primary Axle Powertrain Selector/Hybrid Drive/P0/P0 Motor ==
  n_Upmin IN : Inport
  Torque_P0_sh : Inport  Port=2
  P_max_EM_kW : Inport  Port=3
  P_min_EM_kW : Inport  Port=4
  1-D Lookup Table1 : Lookup_n-D  NumberOfTableDimensions=1  BreakpointsForDimension1=cp.speed_breakpoints_P0  Table=cp.torque_values_P0  InternalRulePriority=Speed  RndMeth=Simplest
  Battery and Operating Strategy Limitation (Recuperation) : Subsystem
  Gain : Gain  Gain=-1
  Min : MinMax  Inputs=2
  Power Calculation : Subsystem
  "Power Calculation " : Subsystem
  Saturation : Saturate  UpperLimit=inf  LowerLimit=0
  SubsysteBattery and Operating Strategy Limitation (Drive)m : Subsystem
  P0_M_Nm_Fahren : Outport
  P_max_EM_P0_kW : Outport  Port=2
  P_min_EM_P0_kW : Outport  Port=3
  P0_M_Nm_Reku : Outport  Port=4
  tag scope: tq_sh_P0_max=global
  wires:
  Power Calculation/1(P_kW) -> P_max_EM_P0_kW/1
  "Power Calculation "/1(P_kW) -> P_min_EM_P0_kW/1
  Saturation/1 -> Min/2
  1-D Lookup Table1/1 -> Gain/1, [tq_sh_P0_max], Min/1  "Torque_ICE_Limit"
  n_Upmin IN/1 -> Battery and Operating Strategy Limitation (Recuperation)/1(Motordrehzahl (1/min)), SubsysteBattery and Operating Strategy Limitation (Drive)m/1(Motordrehzahl (1/min)), 1-D Lookup Table1/1  "Motordrehzahl (1/min)"
  Torque_P0_sh/1 -> Saturation/1
  SubsysteBattery and Operating Strategy Limitation (Drive)m/2(tq_sh_P0_bat_limted) -> P0_M_Nm_Fahren/1, Power Calculation/2(tq_sh_P0_bat_limted)
  Min/1 -> SubsysteBattery and Operating Strategy Limitation (Drive)m/2(tq_sh_P0_limted)  "tq_sh_P0_limted"
  P_max_EM_kW/1 -> SubsysteBattery and Operating Strategy Limitation (Drive)m/3(P_mech_max_kW)
  SubsysteBattery and Operating Strategy Limitation (Drive)m/1(n_Upmin OUT) -> Power Calculation/1(n_Upmin)
  Battery and Operating Strategy Limitation (Recuperation)/2(tq_sh_P0_bat_limted_recu) -> P0_M_Nm_Reku/1, "Power Calculation "/2(tq_sh_P0_bat_limted_recu)
  Gain/1 -> Battery and Operating Strategy Limitation (Recuperation)/2(Torque_Recu_In)
  P_min_EM_kW/1 -> Battery and Operating Strategy Limitation (Recuperation)/3(P_mech_max_kW)
  Battery and Operating Strategy Limitation (Recuperation)/1(n_Upmin OUT) -> "Power Calculation "/1(n_Upmin)

== system Simulation_Fahrmodell_v4_straight_line_v1/Vehicle Dynamics Model /Drivetrain/Primary and Secondary Axle Powertrain Selector/Primary Axle Powertrain Selector/Hybrid Drive/P0/P0 Motor disabled ==
  n_Upmin IN : Inport
  Torque_P0_sh : Inport  Port=2
  P_max_EM_kW : Inport  Port=3
  P_min_EM_kW : Inport  Port=4
  Constant : Constant  Value=0
  Terminator{,1..3} (4 alike) : Terminator
  P0_M_Nm_Fahren : Outport
  P_max_EM_P0_kW : Outport  Port=2
  P_min_EM_P0_kW : Outport  Port=3
  P0_M_Nm_Reku : Outport  Port=4
  wires:
  Constant/1 -> P_min_EM_P0_kW/1, P_max_EM_P0_kW/1, P0_M_Nm_Fahren/1, P0_M_Nm_Reku/1
  n_Upmin IN/1 -> Terminator/1  "Motordrehzahl (1/min)"
  P_max_EM_kW/1 -> Terminator1/1
  P_min_EM_kW/1 -> Terminator2/1
  Torque_P0_sh/1 -> Terminator3/1

== system Simulation_Fahrmodell_v4_straight_line_v1/Vehicle Dynamics Model /Drivetrain/Primary and Secondary Axle Powertrain Selector/Primary Axle Powertrain Selector/Hybrid Drive/P2/P2 Motor ==
  n_Upmin IN : Inport
  Torque_P2_sh : Inport  Port=2
  P_max_EM_kW : Inport  Port=3
  P_min_EM_kW : Inport  Port=4
  1-D Lookup Table1 : Lookup_n-D  NumberOfTableDimensions=1  BreakpointsForDimension1=cp.speed_breakpoints_P2  Table=cp.torque_values_P2  InternalRulePriority=Speed  RndMeth=Simplest
  Battery and Operating Strategy Limitation (Drive) : Subsystem
  Battery and Operating Strategy Limitation (Recuperation) : Subsystem
  Gain : Gain  Gain=-1
  Min : MinMax  Inputs=2
  Power Calculation : Subsystem
  "Power Calculation " : Subsystem
  Saturation : Saturate  UpperLimit=inf  LowerLimit=0
  P2_M_Nm_Fahren : Outport
  P_max_EM_P2_kW : Outport  Port=2
  P_min_EM_P2_kW : Outport  Port=3
  P2_M_Nm_Reku : Outport  Port=4
  tag scope: tq_sh_P2_max=global
  wires:
  Power Calculation/1(P_kW) -> P_max_EM_P2_kW/1  "P_max_EM_P2_kW"
  "Power Calculation "/1(P_kW) -> P_min_EM_P2_kW/1  "P_min_EM_P2_kW"
  Saturation/1 -> Min/2
  1-D Lookup Table1/1 -> Min/1, [tq_sh_P2_max], Gain/1  "Torque_ICE_Limit"
  n_Upmin IN/1 -> Battery and Operating Strategy Limitation (Recuperation)/1(Motordrehzahl (1/min)), Battery and Operating Strategy Limitation (Drive)/1(Motordrehzahl (1/min)), 1-D Lookup Table1/1  "Motordrehzahl (1/min)"
  Torque_P2_sh/1 -> Saturation/1
  Battery and Operating Strategy Limitation (Drive)/2(tq_sh_P2_bat_limted) -> P2_M_Nm_Fahren/1, Power Calculation/2(tq_sh_P2_bat_limted)
  Min/1 -> Battery and Operating Strategy Limitation (Drive)/2(tq_sh_P2_limted)  "tq_sh_P2_limted"
  P_max_EM_kW/1 -> Battery and Operating Strategy Limitation (Drive)/3(P_max_EM_kW)  "P_max_EM_kW"
  Battery and Operating Strategy Limitation (Drive)/1(n_Upmin OUT) -> Power Calculation/1(n_Upmin)
  Battery and Operating Strategy Limitation (Recuperation)/2(tq_sh_P2_bat_limted_recu) -> P2_M_Nm_Reku/1, "Power Calculation "/2(tq_sh_P2_bat_limted_recu)
  Gain/1 -> Battery and Operating Strategy Limitation (Recuperation)/2(Torque_Recu_In)
  P_min_EM_kW/1 -> Battery and Operating Strategy Limitation (Recuperation)/3(P_min_EM_kW)  "P_min_EM_kW"
  Battery and Operating Strategy Limitation (Recuperation)/1(n_Upmin OUT) -> "Power Calculation "/1(n_Upmin)

== system Simulation_Fahrmodell_v4_straight_line_v1/Vehicle Dynamics Model /Drivetrain/Primary and Secondary Axle Powertrain Selector/Primary Axle Powertrain Selector/Hybrid Drive/P2/P2 Motor disabled ==
  n_Upmin IN : Inport
  Torque_P2_sh : Inport  Port=2
  P_max_EM_kW : Inport  Port=3
  P_min_EM_kW : Inport  Port=4
  Constant : Constant  Value=0
  Terminator{,1..3} (4 alike) : Terminator
  P2_M_Nm_Fahren : Outport
  P_max_EM_P2_kW : Outport  Port=2
  P_min_EM_P2_kW : Outport  Port=3
  P2_M_Nm_Reku : Outport  Port=4
  wires:
  Constant/1 -> P_min_EM_P2_kW/1, P_max_EM_P2_kW/1, P2_M_Nm_Fahren/1, P2_M_Nm_Reku/1
  n_Upmin IN/1 -> Terminator/1  "Motordrehzahl (1/min)"
  P_max_EM_kW/1 -> Terminator1/1
  P_min_EM_kW/1 -> Terminator2/1
  Torque_P2_sh/1 -> Terminator3/1

== system Simulation_Fahrmodell_v4_straight_line_v1/Vehicle Dynamics Model /Drivetrain/Primary and Secondary Axle Powertrain Selector/Primary Axle Powertrain Selector/Hybrid Drive/P3/P3 Motor ==
  n_Upmin IN : Inport
  tq_sh_P3_des : Inport  Port=2
  P_max_EM_kW : Inport  Port=3
  P_min_EM_kW : Inport  Port=4
  1-D Lookup Table1 : Lookup_n-D  NumberOfTableDimensions=1  BreakpointsForDimension1=cp.speed_breakpoints_P3  Table=cp.torque_values_P3  InternalRulePriority=Speed  RndMeth=Simplest
  Battery and Operating Strategy Limitation (Drive) : Subsystem
  Battery and Operating Strategy Limitation (Recuperation) : Subsystem
  Gain : Gain  Gain=-1
  Min : MinMax  Inputs=2
  Power Calculation : Subsystem
  "Power Calculation " : Subsystem
  Saturation : Saturate  UpperLimit=inf  LowerLimit=0
  P3_M_Nm_Drive : Outport
  P_max_EM_P3_kW : Outport  Port=2
  P_min_EM_P3_kW : Outport  Port=3
  P3_M_Nm_Recu : Outport  Port=4
  tag scope: tq_sh_P3_max=global
  wires:
  Power Calculation/1(P_max_EM_P3_kW) -> P_max_EM_P3_kW/1
  "Power Calculation "/1(P_kW) -> P_min_EM_P3_kW/1
  Saturation/1 -> Min/2
  1-D Lookup Table1/1 -> [tq_sh_P3_max], Gain/1, Min/1  "tq_sh_P3_lim"
  n_Upmin IN/1 -> 1-D Lookup Table1/1, Battery and Operating Strategy Limitation (Recuperation)/1(n_Upmin IN), Battery and Operating Strategy Limitation (Drive)/1(n_Upmin IN)  "n_Upmin"
  tq_sh_P3_des/1 -> Saturation/1
  Battery and Operating Strategy Limitation (Drive)/2(tq_sh_P3_bat_limted) -> P3_M_Nm_Drive/1, Power Calculation/2(tq_sh_P3_bat_limted)
  Min/1 -> Battery and Operating Strategy Limitation (Drive)/2(tq_sh_P3_limted)  "tq_sh_P3_limted"
  P_max_EM_kW/1 -> Battery and Operating Strategy Limitation (Drive)/3(P_max_EM_kW)
  Battery and Operating Strategy Limitation (Drive)/1(n_Upmin OUT) -> Power Calculation/1(n_Upmin)
  Battery and Operating Strategy Limitation (Recuperation)/2(tq_sh_P3_bat_limted) -> "Power Calculation "/2(tq_sh_P3_bat_limted), P3_M_Nm_Recu/1
  Gain/1 -> Battery and Operating Strategy Limitation (Recuperation)/2(Torque_Recu_In)
  P_min_EM_kW/1 -> Battery and Operating Strategy Limitation (Recuperation)/3(P_mech_max_kW)
  Battery and Operating Strategy Limitation (Recuperation)/1(n_Upmin OUT) -> "Power Calculation "/1(n_Upmin)

== system Simulation_Fahrmodell_v4_straight_line_v1/Vehicle Dynamics Model /Drivetrain/Primary and Secondary Axle Powertrain Selector/Primary Axle Powertrain Selector/Hybrid Drive/P3/P3 Motor disabled ==
  n_Upmin IN : Inport
  tq_sh_P3_des : Inport  Port=2
  P_max_EM_kW : Inport  Port=3
  P_min_EM_kW : Inport  Port=4
  Constant : Constant  Value=0
  Terminator{,1..3} (4 alike) : Terminator
  P3_M_Nm_Drive : Outport
  P_max_EM_P3_kW : Outport  Port=2
  P_min_EM_P3_kW : Outport  Port=3
  P3_M_Nm_Recu : Outport  Port=4
  wires:
  Constant/1 -> P_min_EM_P3_kW/1, P_max_EM_P3_kW/1, P3_M_Nm_Drive/1, P3_M_Nm_Recu/1
  n_Upmin IN/1 -> Terminator/1  "Motordrehzahl (1/min)"
  P_max_EM_kW/1 -> Terminator1/1
  P_min_EM_kW/1 -> Terminator2/1
  tq_sh_P3_des/1 -> Terminator3/1
